simulink library "DYN_GRAV"  (Simulink 8.8)
settings: Solver=ode45  StartTime=0.0  StopTime=10.0  RelTol=1e-3  EnableMultiTasking=on
libraries: LIB_ROT x4, LIB_ENV x3
settings Model: Creator=alger  LastModifiedBy=alger

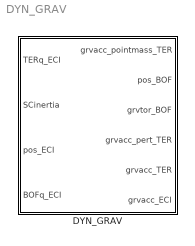
== system DYN_GRAV ==
  DYN_GRAV : Subsystem

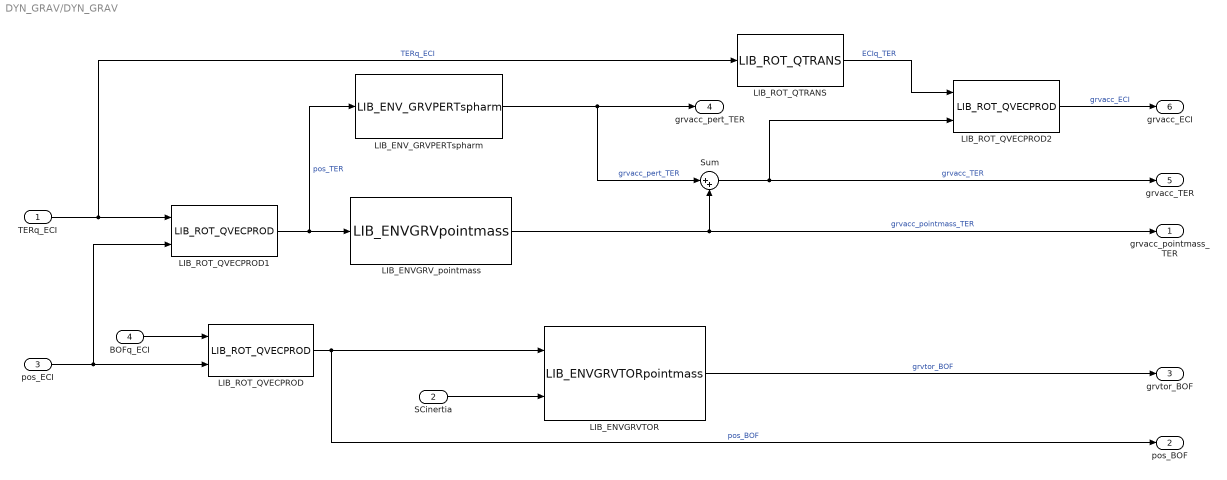
== system DYN_GRAV/DYN_GRAV ==
  TERq_ECI : Inport
  SCinertia : Inport  Port=2
  pos_ECI : Inport  Port=3
  BOFq_ECI : Inport  Port=4
  LIB_ENVGRVTOR : LIB_ENV/LIB_ENVGRVTORpointmass  mu_cst=CONSTANTS_par.mu_earth
  LIB_ENVGRV_pointmass : LIB_ENV/LIB_ENVGRVpointmass  mu_cst=CONSTANTS_par.mu_earth
  LIB_ENV_GRVPERTspharm : LIB_ENV/LIB_ENV_GRVPERTspharm  mu_cst=CONSTANTS_par.mu_earth  re_cst=CONSTANTS_par.r_earth  maxDegree=DYN_GRV_par.max_degree  maxOrder=DYN_GRV_par.max_order  Cnm=DYN_GRV_par.Cnm  Snm=DYN_GRV_par.Snm
  LIB_ROT_QTRANS : LIB_ROT/LIB_ROT_QTRANS
  LIB_ROT_QVECPROD : LIB_ROT/LIB_ROT_QVECPROD
  LIB_ROT_QVECPROD1 : LIB_ROT/LIB_ROT_QVECPROD
  LIB_ROT_QVECPROD2 : LIB_ROT/LIB_ROT_QVECPROD
  Sum : Sum  Inputs=|++
  grvacc_pointmass_TER : Outport
  pos_BOF : Outport  Port=2
  grvtor_BOF : Outport  Port=3
  grvacc_pert_TER : Outport  Port=4
  grvacc_TER : Outport  Port=5
  grvacc_ECI : Outport  Port=6
  wires:
  LIB_ENVGRV_pointmass/1 -> grvacc_pointmass_TER/1, Sum/2  "grvacc_pointmass_TER"
  LIB_ROT_QVECPROD/1 -> pos_BOF/1, LIB_ENVGRVTOR/1  "pos_BOF"
  BOFq_ECI/1 -> LIB_ROT_QVECPROD/1
  LIB_ENVGRVTOR/1 -> grvtor_BOF/1  "grvtor_BOF"
  SCinertia/1 -> LIB_ENVGRVTOR/2
  pos_ECI/1 -> LIB_ROT_QVECPROD1/2, LIB_ROT_QVECPROD/2
  LIB_ROT_QVECPROD1/1 -> LIB_ENV_GRVPERTspharm/1, LIB_ENVGRV_pointmass/1  "pos_TER"
  TERq_ECI/1 -> LIB_ROT_QTRANS/1, LIB_ROT_QVECPROD1/1  "TERq_ECI"
  LIB_ENV_GRVPERTspharm/1 -> Sum/1, grvacc_pert_TER/1  "grvacc_pert_TER"
  Sum/1 -> LIB_ROT_QVECPROD2/2, grvacc_TER/1  "grvacc_TER"
  LIB_ROT_QVECPROD2/1 -> grvacc_ECI/1  "grvacc_ECI"
  LIB_ROT_QTRANS/1 -> LIB_ROT_QVECPROD2/1  "ECIq_TER"
